simulink model "untitled1"  (R2019b)
settings: Solver=VariableStepAuto  StartTime=0.0  StopTime=100.0  RelTol=1e-3
values from neighbouring files (symbols this model uses):
  A = [0 1 0; 0 0 1; -1 -8 -80]    [init.m]
  b = [1; 0; 0]    [init.m]
  cT = [1 0 0]    [init.m]
libraries: cstblocks x1

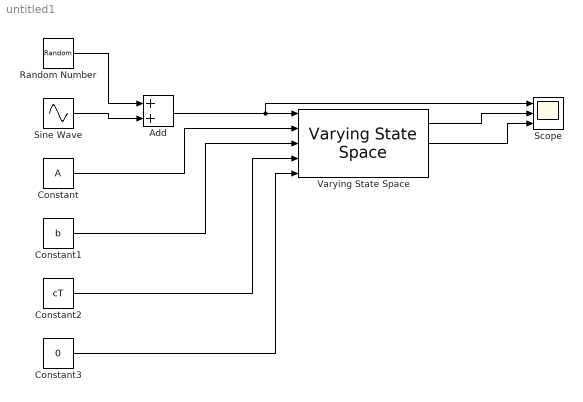
== system untitled1 ==
  Add : Sum
  Constant : Constant  Value=A  VectorParams1D=off
  Constant1 : Constant  Value=b  VectorParams1D=off
  Constant2 : Constant  Value=cT  VectorParams1D=off
  Constant3 : Constant  Value=0
  Random Number : RandomNumber  Variance=0.2  SampleTime=0.1
  Scope : Scope  NumInputPorts=3
  Sine Wave : Sin  Frequency=0.1  SampleTime=0
  Varying State Space : cstblocks/Linear Parameter Varying/Varying State Space  x0=0  xNames=''  OutputX=on  OutputDX=on
  wires:
  Add/1 -> Scope/1, Varying State Space/1
  Sine Wave/1 -> Add/2
  Random Number/1 -> Add/1
  Constant/1 -> Varying State Space/2
  Constant1/1 -> Varying State Space/3
  Constant2/1 -> Varying State Space/4
  Constant3/1 -> Varying State Space/5
  Varying State Space/1 -> Scope/2
  Varying State Space/2 -> Scope/3
